simulink model "s_mbd_02_04"  (R2020b)
settings: Solver=ode4  StartTime=0.0  StopTime=Endtime  FixedStep=0.1  RelTol=1e-3
values from neighbouring files (symbols this model uses):
  C = pi*D^2/4    (= 0.196349540849)    [m_mbd_02_04.m]    (also in s_heatbalance.m = 4200)
  R = 500    [m_mbd_02_04.m]    (also in s_heatbalance.m = 0.1)
settings Model: Creator=005274  LastModifiedBy=005274

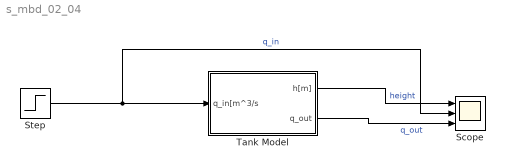
== system s_mbd_02_04 ==
  Scope : Scope  NumInputPorts=3
  Step : Step  SampleTime=0
  Tank Model : Subsystem
  wires:
  Step/1 -> Tank Model/1(q_in[m^3/s), Scope/2  "q_in"
  Tank Model/1(h[m]) -> Scope/1  "height"
  Tank Model/2(q_out) -> Scope/3  "q_out"

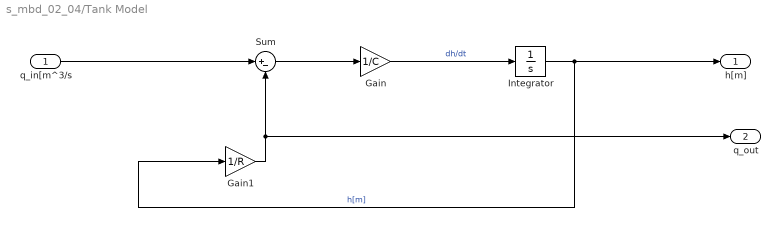
== system s_mbd_02_04/Tank Model ==
  q_in[m^3/s : Inport
  Gain : Gain  Gain=1/C
  Gain1 : Gain  Gain=1/R
  Integrator : Integrator
  Sum : Sum  Inputs=|+-
  h[m] : Outport
  q_out : Outport  Port=2
  wires:
  Gain/1 -> Integrator/1  "dh/dt"
  Integrator/1 -> h[m]/1, Gain1/1  "h[m]"
  Gain1/1 -> q_out/1, Sum/2
  q_in[m^3/s/1 -> Sum/1
  Sum/1 -> Gain/1
